simulink model "DOFTest"  (R2024b)
settings: Solver=VariableStepAuto  StartTime=0.0  StopTime=10.0  RelTol=1e-3
settings Model: Creator=jebid  LastModifiedBy=jebid

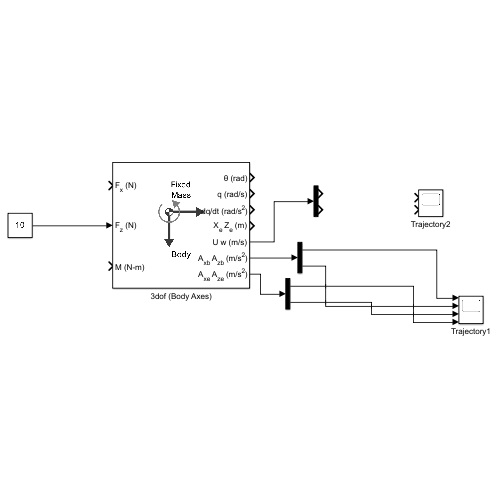
[thumbnail: Simulink's stored preview of the top-level diagram]
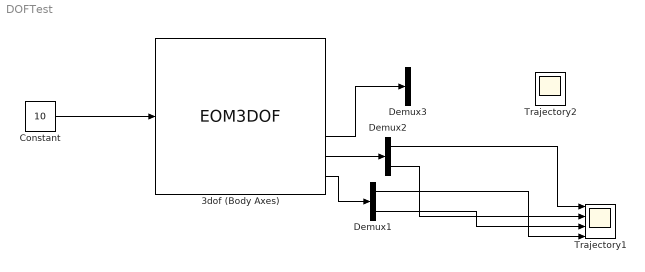
== system DOFTest ==
  3dof (Body Axes) : EOM3DOF  v_ini=0  theta_ini=0.25  mass=0.5  Iyy=0.05  g=0  abi_flag=on
  Constant : Constant  Value=10
  Demux1 : Demux  Outputs=2
  Demux2 : Demux  Outputs=2
  Demux3 : Demux  Outputs=2
  Trajectory1 : Scope  NumInputPorts=4
  Trajectory2 : Scope  NumInputPorts=2
  wires:
  Constant/1 -> 3dof (Body Axes)/2
  Demux1/1 -> Trajectory1/4
  Demux2/1 -> Trajectory1/1
  3dof (Body Axes)/6 -> Demux2/1
  3dof (Body Axes)/7 -> Demux1/1
  Demux1/2 -> Trajectory1/3
  Demux2/2 -> Trajectory1/2
  3dof (Body Axes)/5 -> Demux3/1
